simulink model "tank_sim"  (R2020b)
settings: Solver=VariableStepAuto  StartTime=0.0  StopTime=1000  RelTol=1e-3
values from neighbouring files (symbols this model uses):
  A = [-b/J, Kt/J; -Ke/l, -r/l]    [dcmotor.m]    (also in makedcmotorparams.m; tanks.m = [-1/Ti(1, Area(1))            0;      Area(1)/Area(2)/Ti(h0,)
  a = (2.5e-2)^2*60    (= 0.0375)    [tanks.m]
  Area = [1 1]    [tanks.m]
  B = [0; 1/l]    [dcmotor.m]    (also in makedcmotorparams.m; tanks.m = [1/Area(1); 0])
  C = [1, 1]    [dcmotor.m]    (also in makedcmotorparams.m; tanks.m = [0 1])
  E = [0; -1/Area(2)]    [tanks.m]
  g = 9.81    [tanks.m]
  L = place(Ad', Cd', [0.6, 0.5]).'    [dcmotor.m]    (also in makedcmotorparams.m = place(Ad', Cd', [0.6, 0]).'; tanks.m = place(A', C', [-100 -2])')
libraries: LinSysLib x1
settings Model: Creator=angelo  LastModifiedBy=angelo

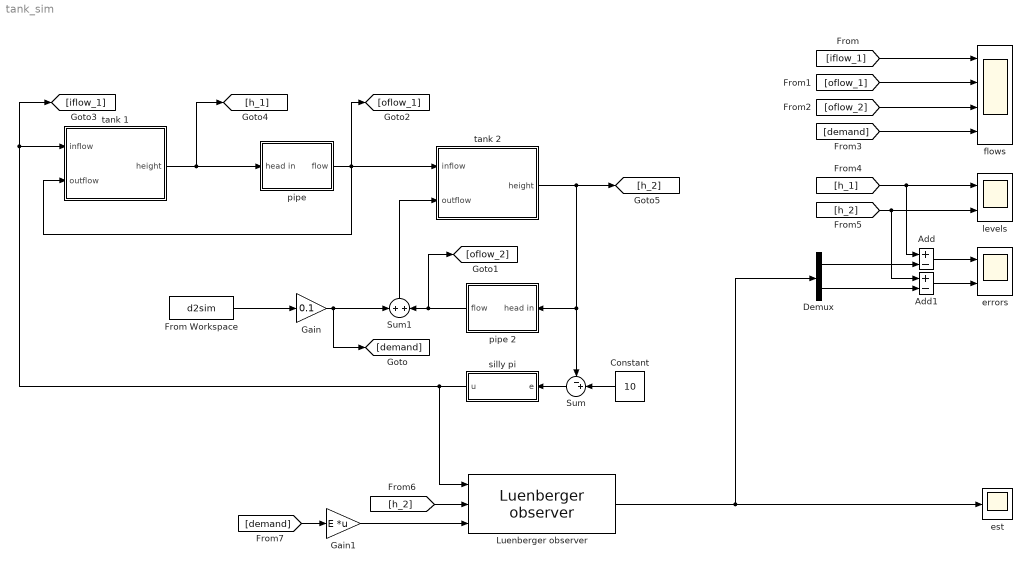
== system tank_sim ==
  Add : Sum  Inputs=+-
  Add1 : Sum  Inputs=+-
  Constant : Constant  Value=10
  Demux : Demux  Outputs=2
  From Workspace : FromWorkspace  VariableName=d2sim  OutDataTypeStr=double  SampleTime=.1  Interpolate=off  OutputAfterFinalValue=Cyclic repetition
  Gain : Gain  Gain=0.1
  Gain1 : Gain  Gain=E  Multiplication=Matrix(K*u)
  Luenberger observer : LinSysLib/Continuous time/Luenberger observer  A=A  B=B  C=C  D=0  hatx0=zeros(2,1)  L=L
  Sum : Sum  Inputs=-+|
  Sum1 : Sum  Inputs=+|+
  errors : Scope  NumInputPorts=2
  est : Scope
  flows : Scope  NumInputPorts=4
  levels : Scope  NumInputPorts=2
  pipe : Subsystem  mask{flowCoeff=1, pipeArea=a, g=g}
      mask prompts: flowCoeff "flow coefficient"; pipeArea "pipe area"; g "gravity acceleration"
  pipe 2 : Subsystem  mask{flowCoeff=1, pipeArea=a, g=g}
      mask prompts: flowCoeff "flow coefficient"; pipeArea "pipe area"; g "gravity acceleration"
  silly pi : Subsystem
  tank 1 : Subsystem  mask{area=Area(1), h0=10}
      mask prompts: area "Area [m^2]"; h0 "Initial level [m]"
  tank 2 : Subsystem  mask{area=Area(2), h0=2}
      mask prompts: area "Area [m^2]"; h0 "Initial level [m]"
  wires:
  tank 2/1(height) -> [h_2], Sum/1, pipe 2/1(head in)
  tank 1/1(height) -> [h_1], pipe/1(head in)
  pipe/1(flow) -> [oflow_1], tank 2/1(inflow), tank 1/2(outflow)
  Constant/1 -> Sum/2
  Sum/1 -> silly pi/1(e)
  silly pi/1(u) -> Luenberger observer/1, [iflow_1], tank 1/1(inflow)
  pipe 2/1(flow) -> [oflow_2], Sum1/2
  From Workspace/1 -> Gain/1
  Sum1/1 -> tank 2/2(outflow)
  Gain/1 -> [demand], Sum1/1
  [demand] -> flows/4
  [oflow_2] -> flows/3
  [oflow_1] -> flows/2
  [iflow_1] -> flows/1
  [h_2] -> Add1/1, levels/2
  [h_2] -> Luenberger observer/2
  Gain1/1 -> Luenberger observer/3
  Luenberger observer/1 -> est/1, Demux/1
  [h_1] -> Add/1, levels/1
  Demux/1 -> Add/2
  Demux/2 -> Add1/2
  Add/1 -> errors/1
  Add1/1 -> errors/2
  [demand] -> Gain1/1

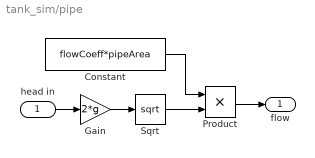
== system tank_sim/pipe ==
  head in : Inport
  Constant : Constant  Value=flowCoeff*pipeArea
  Gain : Gain  Gain=2*g
  Product : Product
  Sqrt : Sqrt  OutputSignalType=real  SaturateOnIntegerOverflow=on
  flow : Outport  VectorParamsAs1DForOutWhenUnconnected=off
  wires:
  Constant/1 -> Product/1
  Gain/1 -> Sqrt/1
  head in/1 -> Gain/1
  Product/1 -> flow/1
  Sqrt/1 -> Product/2

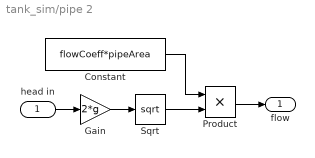
== system tank_sim/pipe 2 ==
  head in : Inport
  Constant : Constant  Value=flowCoeff*pipeArea
  Gain : Gain  Gain=2*g
  Product : Product
  Sqrt : Sqrt  OutputSignalType=real  SaturateOnIntegerOverflow=on
  flow : Outport  VectorParamsAs1DForOutWhenUnconnected=off
  wires:
  Sqrt/1 -> Product/2
  Product/1 -> flow/1
  head in/1 -> Gain/1
  Gain/1 -> Sqrt/1
  Constant/1 -> Product/1

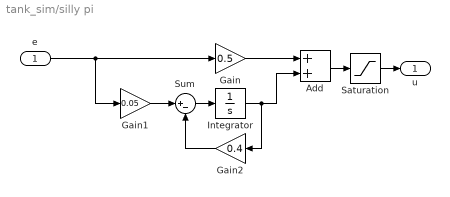
== system tank_sim/silly pi ==
  e : Inport
  Add : Sum
  Gain : Gain  Gain=0.5
  Gain1 : Gain  Gain=0.05
  Gain2 : Gain  Gain=0.4
  Integrator : Integrator
  Saturation : Saturate  UpperLimit=Inf  LowerLimit=0
  Sum : Sum  Inputs=|+-
  u : Outport  VectorParamsAs1DForOutWhenUnconnected=off
  wires:
  Integrator/1 -> Gain2/1, Add/2
  Gain/1 -> Add/1
  Gain1/1 -> Sum/1
  Add/1 -> Saturation/1
  e/1 -> Gain1/1, Gain/1
  Saturation/1 -> u/1
  Sum/1 -> Integrator/1
  Gain2/1 -> Sum/2

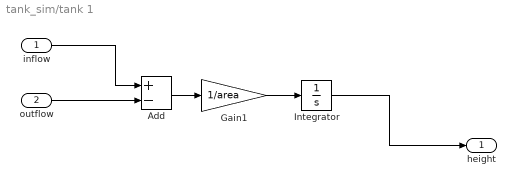
== system tank_sim/tank 1 ==
  inflow : Inport
  outflow : Inport  Port=2
  Add : Sum  Inputs=+-
  Gain1 : Gain  Gain=1/area
  Integrator : Integrator  InitialCondition=h0  LimitOutput=on  LowerSaturationLimit=0
  height : Outport  VectorParamsAs1DForOutWhenUnconnected=off
  wires:
  Integrator/1 -> height/1
  Gain1/1 -> Integrator/1
  Add/1 -> Gain1/1
  inflow/1 -> Add/1
  outflow/1 -> Add/2

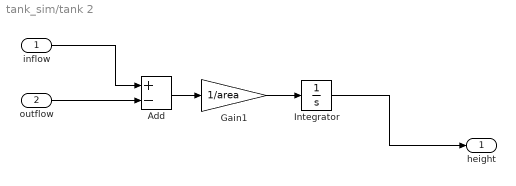
== system tank_sim/tank 2 ==
  inflow : Inport
  outflow : Inport  Port=2
  Add : Sum  Inputs=+-
  Gain1 : Gain  Gain=1/area
  Integrator : Integrator  InitialCondition=h0  LimitOutput=on  LowerSaturationLimit=0
  height : Outport  VectorParamsAs1DForOutWhenUnconnected=off
  wires:
  outflow/1 -> Add/2
  inflow/1 -> Add/1
  Add/1 -> Gain1/1
  Gain1/1 -> Integrator/1
  Integrator/1 -> height/1
